simulink model "Marine_LocoMotive_UAV"  (R2018a)
settings: Solver=ode4  StartTime=0.0  StopTime=80  FixedStep=T  RelTol=1e-3
values from neighbouring files (symbols this model uses):
  a_11 = 0.05*m_b    (= 0.625)    [Marine_LocoMotive_UAV.m]
  a_33 = m_b    (= 12.5)    [Marine_LocoMotive_UAV.m]
  A_w = 1*1.5/2    (= 0.75)    [Marine_LocoMotive_UAV.m]
  A_w2 = 1*0.27/2    (= 0.135)    [Marine_LocoMotive_UAV.m]
  Ac = 0.0331    [Marine_LocoMotive_UAV.m]
  alpha_bar = pi/4    (= 0.785398163397)    [Marine_LocoMotive_UAV.m]
  Am = sysd.denominator{1}    [Marine_LocoMotive_UAV.m]
  Am1_LPF = sysd.denominator{1}    [Marine_LocoMotive_UAV.m]
  Am2_LPF = sysd.denominator{1}    [Marine_LocoMotive_UAV.m]
  Am_asw_LPF = sysd.denominator{1}    [Marine_LocoMotive_UAV.m]
  Am_coup_LPF = sysd.denominator{1}    [Marine_LocoMotive_UAV.m]
  Am_rdeL_LPF = sysd.denominator{1}    [Marine_LocoMotive_UAV.m]
  Am_reL_LPF = sysd.denominator{1}    [Marine_LocoMotive_UAV.m]
  Am_rref20_LPF = sysd.denominator{1}    [Marine_LocoMotive_UAV.m]
  Am_rref_LPF = sysd.denominator{1}    [Marine_LocoMotive_UAV.m]
  AmAlpha_LPF = sysd.denominator{1}    [Marine_LocoMotive_UAV.m]
  Amp_sf = 3    [Marine_LocoMotive_UAV.m]
  AmV_LPF = sysd.denominator{1}    [Marine_LocoMotive_UAV.m]
  AmZ_LPF = sysd.denominator{1}    [Marine_LocoMotive_UAV.m]
  b_11 = 0    [Marine_LocoMotive_UAV.m]
  b_33 = 2*m_b*omega_h    (= 27.5578302946)    [Marine_LocoMotive_UAV.m]
  Bm = sysd.numerator{1}    [Marine_LocoMotive_UAV.m]
  Bm1_LPF = sysd.numerator{1}    [Marine_LocoMotive_UAV.m]
  Bm2_LPF = sysd.numerator{1}    [Marine_LocoMotive_UAV.m]
  Bm_asw_LPF = sysd.numerator{1}    [Marine_LocoMotive_UAV.m]
  Bm_coup_LPF = sysd.numerator{1}    [Marine_LocoMotive_UAV.m]
  Bm_rdeL_LPF = sysd.numerator{1}    [Marine_LocoMotive_UAV.m]
  Bm_reL_LPF = sysd.numerator{1}    [Marine_LocoMotive_UAV.m]
  Bm_rref20_LPF = sysd.numerator{1}    [Marine_LocoMotive_UAV.m]
  Bm_rref_LPF = sysd.numerator{1}    [Marine_LocoMotive_UAV.m]
  BmAlpha_LPF = sysd.numerator{1}    [Marine_LocoMotive_UAV.m]
  BmV_LPF = sysd.numerator{1}    [Marine_LocoMotive_UAV.m]
  BmZ_LPF = sysd.numerator{1}    [Marine_LocoMotive_UAV.m]
  C_S = [5;9]*10^-3    [Marine_LocoMotive_UAV.m]
  Cd_u = 0.2    [Marine_LocoMotive_UAV.m]
  D_x = b_11 + D_s(1)    [Marine_LocoMotive_UAV.m]
  D_z = b_33 + D_s(2)    [Marine_LocoMotive_UAV.m]
  dc_M_p = 6.7    [Marine_LocoMotive_UAV.m]
  Delta_h = (A_im/A_b-0.5)*h_b    (= -0.0625)    [Marine_LocoMotive_UAV.m]
  eps_V = 0.1    [Marine_LocoMotive_UAV.m]
  epsilon_1 = 5    [Marine_LocoMotive_UAV.m]
  epsilon_e_u1 = 0.05    [Marine_LocoMotive_UAV.m]
  epsilon_w = 0    [Marine_LocoMotive_UAV.m]
  epsilon_w2 = pi    (= 3.14159265359)    [Marine_LocoMotive_UAV.m]
  g = 9.81    [Marine_LocoMotive_UAV.m]
  gamma_d_p = (2*0.3/0.03*2*0.2*12/4)/10    (= 2.4)    [Marine_LocoMotive_UAV.m]
  H = 10    [Marine_LocoMotive_UAV.m]
  h_b = 0.25    [Marine_LocoMotive_UAV.m]
  J_b = m_b*h_b*l_b/12    (= 0.208333333333)    [Marine_LocoMotive_UAV.m]
  J_u = 0.03    [Marine_LocoMotive_UAV.m]
  K = 40    [Marine_LocoMotive_UAV.m]
  k3 = 24    [Marine_LocoMotive_UAV.m]
  k4 = 0.8    [Marine_LocoMotive_UAV.m]
  k_w = omega_w^2/g    (= 0.123862835563)    [Marine_LocoMotive_UAV.m]
  k_w2 = omega_w2^2/g    (= 0.447144836384)    [Marine_LocoMotive_UAV.m]
  kd_a = 5.6    [Marine_LocoMotive_UAV.m]
  kd_r = 19.5    [Marine_LocoMotive_UAV.m]
  kd_t = 10    [Marine_LocoMotive_UAV.m]
  kd_x = 5    [Marine_LocoMotive_UAV.m]
  kd_z = 2    [Marine_LocoMotive_UAV.m]
  ki_a = 1.6    [Marine_LocoMotive_UAV.m]
  ki_r = 9    [Marine_LocoMotive_UAV.m]
  ki_T = 12    [Marine_LocoMotive_UAV.m]
  ki_x = 1.2    [Marine_LocoMotive_UAV.m]
  ki_z = 1    [Marine_LocoMotive_UAV.m]
  kp_a = 9.6    [Marine_LocoMotive_UAV.m]
  kp_r = 45    [Marine_LocoMotive_UAV.m]
  kp_t = 20    [Marine_LocoMotive_UAV.m]
  kp_T = 25    [Marine_LocoMotive_UAV.m]
  kp_x = 7    [Marine_LocoMotive_UAV.m]
  kp_z = 3    [Marine_LocoMotive_UAV.m]
  L = 0.2    [Marine_LocoMotive_UAV.m]
  l_b = 0.8    [Marine_LocoMotive_UAV.m]
  Lc_0 = 7    [Marine_LocoMotive_UAV.m]
  LIMIT_CMD_PITCH = 45*pi/180    (= 0.785398163397)    [Marine_LocoMotive_UAV.m]
  LIMIT_uCMD_HEIGHT = 3.5*K    (= 140)    [Marine_LocoMotive_UAV.m]
  m_b = rho_w*Vol_b/4    (= 12.5)    [Marine_LocoMotive_UAV.m]
  m_u = 1.8    [Marine_LocoMotive_UAV.m]
  min_sf = 5    [Marine_LocoMotive_UAV.m]
  nu_w = 1.787*10^-6    (= 1.787e-06)    [Marine_LocoMotive_UAV.m]
  omega_w = 2*pi/T_w    (= 1.10231321179)    [Marine_LocoMotive_UAV.m]
  omega_w2 = 2*pi/T_w2    (= 2.09439510239)    [Marine_LocoMotive_UAV.m]
  r_0 = sqrt( (X0_b(1) - X0_u(1))^2 +(X0_b(2) - X0_u(2))^2 )    [Marine_LocoMotive_UAV.m]
  r_bar = Lc_0-0.3    (= 6.7)    [Marine_LocoMotive_UAV.m]
  r_min = (zu_bar-H)-0.2    [Marine_LocoMotive_UAV.m]
  rho_a = 1.225    [Marine_LocoMotive_UAV.m]
  rho_w = 1000    [Marine_LocoMotive_UAV.m]
  T = 1/500    (= 0.002)    [Marine_LocoMotive_UAV.m]
  T_init = 10    [Marine_LocoMotive_UAV.m]
  Theta0 = 0*atan2(V_bar*D_x*cos(alpha_bar_0),V_bar*D_x*sin(alpha_bar_0)+m_u*g*cos(alpha_bar_0))    [Marine_LocoMotive_UAV.m]
  u_s = w_dir*A_w^2*omega_w*k_w*exp(2*k_w*(-Delta_h/2))    [Marine_LocoMotive_UAV.m]
  u_s2 = w_dir2*A_w2^2*omega_w2*k_w2*exp(2*k_w2*(-Delta_h/2))    [Marine_LocoMotive_UAV.m]
  u_t = -1*0.5*1    (= -0.5)    [Marine_LocoMotive_UAV.m]
  u_w = 0*0.2    (= 0)    [Marine_LocoMotive_UAV.m]
  V0_b = [u_t+u_w+u_s+v_x_w, v_z_w]    [Marine_LocoMotive_UAV.m]
  V0_u = [0 0]    [Marine_LocoMotive_UAV.m]
  V_bar = 4    [Marine_LocoMotive_UAV.m]
  Vol_b = A_b*l_b    (= 0.05)    [Marine_LocoMotive_UAV.m]
  w_dir = 1    [Marine_LocoMotive_UAV.m]
  w_dir2 = 1    [Marine_LocoMotive_UAV.m]
  X0_b = [0,H-Delta_h]    [Marine_LocoMotive_UAV.m]
  X0_u = X0_b + [3 3]    [Marine_LocoMotive_UAV.m]
  zu_bar = X0_b(2) + Lc_0*sin(alpha_bar_0)    [Marine_LocoMotive_UAV.m]
undefined symbols (not defined in the file or in its folder): Am_HPF, Am_LPF, Am_LPF2, an1, an1_v, an2, an3, Bm_HPF, Bm_LPF, Bm_LPF2, bn1, bn1_v, bn2, bn3, DiscIntNeverNeededParam, F, Light, magnitude, MIL, OMEGA_FILTER_OUTER, R_b, Tc, Tg, Tn, Ts, Tsc, Tz, X_GPS_offset
libraries: simulink x50, simulink_extras x9, aerolibwind2 x2
(part 2 of 6)

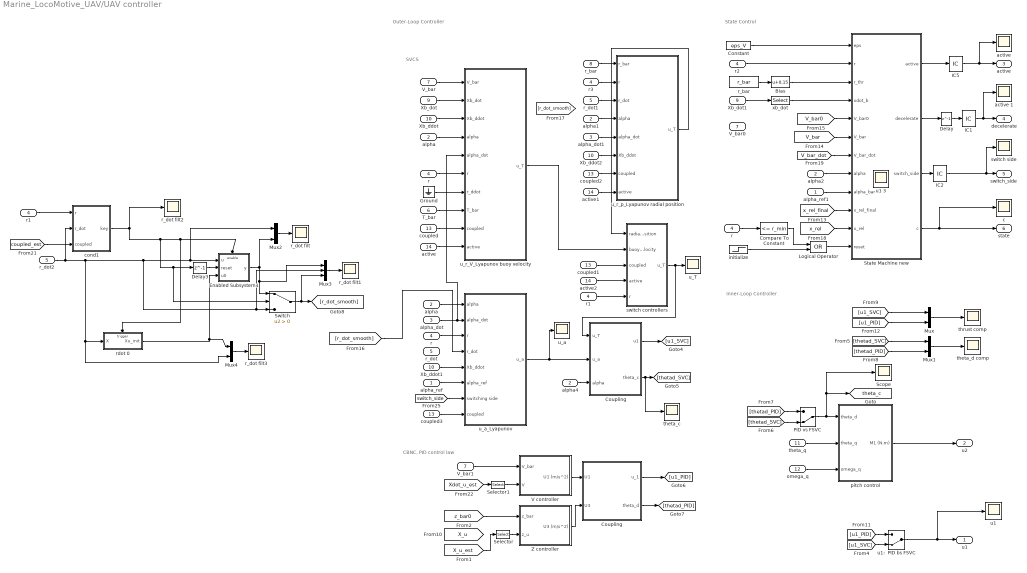
== system Marine_LocoMotive_UAV/UAV controller ==
  note: State Control
  note: Inner-Loop Controller
  note: Outer-Loop Controller
  note: CBNC, PID control law
  note: SVCS
  alpha_ref : Inport
  alpha : Inport  Port=2
  alpha_dot : Inport  Port=3
  r : Inport  Port=4
  r_dot : Inport  Port=5
  T_bar : Inport  Port=6
  V_bar : Inport  Port=7
  r_bar : Inport  Port=8
  Xb_dot : Inport  Port=9
  Xb_ddot : Inport  Port=10
  theta_q : Inport  Port=11
  omega_q : Inport  Port=12
  coupled : Inport  Port=13
  active : Inport  Port=14
  " active " : Scope
  " active 1" : Scope
  " c " : Scope
  " r" : InportShadow  Port=4
  " r1" : InportShadow  Port=4
  Bias : Bias  Bias=0.15
  Compare To Constant : simulink/Logic and Bit Operations/Compare To Constant  relop=<=  const=r_min  OutDataTypeStr=boolean
  Constant : Constant  Value=eps_V
  Coupling : Subsystem
  "Coupling " : Subsystem
  Delay : Delay  DelayLength=1  InitialCondition=0
  Delay3 : Delay  DelayLength=1  InitialCondition=0
  Enabled Subsystem1 : Subsystem  TreatAsAtomicUnit=on
  Ground : Ground
  IC1 : InitialCondition  Value=0
  IC2 : InitialCondition  Value=0
  IC5 : InitialCondition  Value=0
  Logical Operator : Logic  Operator=OR  AllPortsSameDT=off  OutDataTypeStr=boolean
  Mux{,1..2,4} (4 alike) : Mux  Inputs=2
  Mux3 : Mux  Inputs=3
  PID vs FSVC : ManualSwitch  CurrentSetting=0
  Scope : Scope
  Selector : Selector  InputPortWidth=2  IndexOptions=Index vector (dialog)  Indices=2  OutputSizes=1
  Selector1 : Selector  InputPortWidth=2  IndexOptions=Index vector (dialog)  Indices=1  OutputSizes=1
  State Machine new : MATLAB Function  TreatAsAtomicUnit=on
  Switch : Switch  Criteria=u2 > Threshold
  V controller : Subsystem
  V_bar0 : InportShadow  Port=7
  V_bar1 : InportShadow  Port=7
  Xb_ddot1 : InportShadow  Port=10
  Xb_ddot2 : InportShadow  Port=10
  Xb_dot1 : InportShadow  Port=9
  Z controller : Subsystem
  active1 : InportShadow  Port=14
  active2 : InportShadow  Port=14
  "alpha " : InportShadow  Port=2
  alpha1 : InportShadow  Port=2
  alpha2 : InportShadow  Port=2
  alpha4 : InportShadow  Port=2
  alpha_dot1 : InportShadow  Port=3
  alpha_ref1 : InportShadow
  cond1 : Subsystem
  coupled1 : InportShadow  Port=13
  coupled2 : InportShadow  Port=13
  coupled3 : InportShadow  Port=13
  initialize : Step  Time=T_init  Before=1  After=0  SampleTime=0
  pitch control : Subsystem
  "r " : InportShadow  Port=4
  r1 : InportShadow  Port=4
  r2 : InportShadow  Port=4
  r3 : InportShadow  Port=4
  "r_bar " : Constant  Value=r_bar
  r_dot filt{,1..3} (4 alike) : Scope
  r_dot1 : InportShadow  Port=5
  r_dot2 : InportShadow  Port=5
  rdot 0 : Subsystem  TreatAsAtomicUnit=on
  switch controllers : Subsystem
  "switch side  " : Scope
  "theta_c " : Scope
  theta_d comp : Scope
  thrust comp : Scope
  "u1 " : Scope
  u1 3 : Scope
  u1:  PID bs FSVC : ManualSwitch  CurrentSetting=0
  u_T : Scope
  u_a : Scope
  u_a_Lyapunov : Subsystem
  u_r_V_Lyapunov buoy velocity : Subsystem
  u_r_p_Lyapunov radial position : Subsystem
  xb_dot : Selector  InputPortWidth=2  IndexOptions=Index vector (dialog)  Indices=1  OutputSizes=1
  u1 : Outport
  u2 : Outport  Port=2
  " active" : Outport  Port=3
  " decelerate" : Outport  Port=4
  " switch_side" : Outport  Port=5
  state : Outport  Port=6
  tag scope: theta_c=global
  wires:
  theta_q/1 -> pitch control/2(theta_q)
  omega_q/1 -> pitch control/3(omega_q)
  pitch control/1(M1 (N.m)) -> u2/1
  alpha4/1 -> "Coupling "/3(alpha)
  PID vs FSVC/1 -> Scope/1, [theta_c], pitch control/1(theta_d)
  u1:  PID bs FSVC/1 -> "u1 "/1, u1/1
  alpha/1 -> u_r_V_Lyapunov buoy velocity/4(alpha)
  T_bar/1 -> u_r_V_Lyapunov buoy velocity/8(T_bar)
  V_bar/1 -> u_r_V_Lyapunov buoy velocity/1(V_bar)
  Xb_dot/1 -> u_r_V_Lyapunov buoy velocity/2(Xb_dot)
  Xb_ddot/1 -> u_r_V_Lyapunov buoy velocity/3(Xb_ddot)
  "alpha "/1 -> u_a_Lyapunov/1(alpha)
  Xb_ddot1/1 -> u_a_Lyapunov/5(Xb_ddot)
  alpha_ref/1 -> u_a_Lyapunov/6(alpha_ref)
  alpha_dot/1 -> u_r_V_Lyapunov buoy velocity/5(alpha_dot), u_a_Lyapunov/2("alpha_dot ")
  [z_bar0] -> Z controller/1(z_bar)
  Selector/1 -> Z controller/2(z_u)
  [X_u_est] -> Selector/1
  V_bar1/1 -> V controller/1(V_bar)
  [Xdot_u_est] -> Selector1/1
  Selector1/1 -> V controller/2(V)
  V controller/1(U1 (m/s^2)) -> Coupling/1(U1)
  Z controller/1(U3 (m/s^2)) -> Coupling/2(U3)
  Mux/1 -> thrust comp/1
  Mux1/1 -> theta_d comp/1
  [thetad_SVC] -> Mux1/1
  [u1_SVC] -> u1:  PID bs FSVC/2
  u_a_Lyapunov/1(u_a) -> u_a/1, "Coupling "/2(u_a)
  Xb_dot1/1 -> xb_dot/1
  [V_bar0] -> State Machine new/5(V_bar0)
  xb_dot/1 -> State Machine new/4(xdot_b)
  Constant/1 -> State Machine new/1(eps)
  State Machine new/1(active) -> IC5/1
  State Machine new/4(c) -> state/1, " c "/1
  IC5/1 -> " active "/1, " active"/1
  Coupling/1(u_1) -> [u1_PID]
  Coupling/2(theta_d) -> [thetad_PID]
  "Coupling "/1(u1) -> [u1_SVC]
  [thetad_SVC] -> PID vs FSVC/2
  [thetad_PID] -> PID vs FSVC/1
  [thetad_PID] -> Mux1/2
  [u1_SVC] -> Mux/1
  [u1_PID] -> u1:  PID bs FSVC/1
  [u1_PID] -> Mux/2
  "Coupling "/2(theta_c) -> "theta_c "/1, [thetad_SVC]
  r_bar/1 -> u_r_p_Lyapunov radial position/1("r_bar ")
  r/1 -> Compare To Constant/1
  Compare To Constant/1 -> Logical Operator/1
  initialize/1 -> Logical Operator/2
  active/1 -> u_r_V_Lyapunov buoy velocity/10(active)
  coupled/1 -> u_r_V_Lyapunov buoy velocity/9(coupled)
  Ground/1 -> u_r_V_Lyapunov buoy velocity/7(r_ddot)
  [r_dot_smooth] -> u_a_Lyapunov/4(r_dot)
  "r "/1 -> u_r_V_Lyapunov buoy velocity/6(r)
  " r"/1 -> u_a_Lyapunov/3(r)
  r3/1 -> u_r_p_Lyapunov radial position/2(r)
  r_dot1/1 -> u_r_p_Lyapunov radial position/3(r_dot)
  alpha1/1 -> u_r_p_Lyapunov radial position/4(alpha)
  alpha_dot1/1 -> u_r_p_Lyapunov radial position/5(alpha_dot)
  Xb_ddot2/1 -> u_r_p_Lyapunov radial position/6(Xb_ddot)
  active1/1 -> u_r_p_Lyapunov radial position/8(active)
  "r_bar "/1 -> Bias/1
  coupled2/1 -> u_r_p_Lyapunov radial position/7(coupled)
  switch controllers/1(u_T) -> "Coupling "/1(u_T), u_T/1
  u_r_V_Lyapunov buoy velocity/1(u_T) -> switch controllers/2(buoy velocity)
  coupled1/1 -> switch controllers/3(coupled)
  active2/1 -> switch controllers/4(active)
  u_r_p_Lyapunov radial position/1(u_T) -> switch controllers/1(radial position)
  State Machine new/2(decelerate) -> Delay/1
  IC1/1 -> " active 1"/1, " decelerate"/1
  alpha_ref1/1 -> State Machine new/9(alpha_bar)
  alpha2/1 -> State Machine new/8(alpha)
  State Machine new/3(switch_side) -> IC2/1
  IC2/1 -> "switch side  "/1, " switch_side"/1
  Logical Operator/1 -> State Machine new/12(reset)
  r1/1 -> switch controllers/5(r)
  [x_rel_final] -> State Machine new/10(x_rel_final)
  [switch_side] -> u_a_Lyapunov/7(switching side)
  Mux2/1 -> r_dot filt/1
  Enabled Subsystem1/1(y) -> Mux2/2, Mux3/1, Switch/1
  Switch/1 -> Mux3/3, [r_dot_smooth]
  Mux3/1 -> r_dot filt1/1
  [coupled_est] -> cond1/3(coupled)
  coupled3/1 -> u_a_Lyapunov/8(coupled)
  r_dot2/1 -> cond1/2(r_dot), Enabled Subsystem1/1(u), Mux2/1, Mux3/2, Switch/3, rdot 0/1(X), Mux4/2
  Mux4/1 -> r_dot filt3/1
  rdot 0/1(Xu_init) -> Mux4/1, Enabled Subsystem1/3(u0)
  " r1"/1 -> cond1/1(r)
  cond1/1(key) -> Delay3/1, Switch/2, rdot 0/Trigger, Enabled Subsystem1/Enable, r_dot filt2/1
  Delay3/1 -> Enabled Subsystem1/2(reset)
  [x_rel] -> State Machine new/11(x_rel)
  [V_bar] -> State Machine new/6(V_bar)
  Bias/1 -> State Machine new/3(r_thr)
  [V_bar_dot] -> State Machine new/7(V_bar_dot)
  Delay/1 -> IC1/1
  r2/1 -> State Machine new/2(r)

== system Marine_LocoMotive_UAV/Wind model ==
  Bias : Bias  Bias=0.05
  Discrete Wind Gust Model : aerolibwind2/Discrete Wind Gust Model  units=Metric (MKS)  Gx=on  Gy=off  Gz=off  t_0=1  d_m=[1 1 80]  v_m=V_w
      settings: SourceProductName=Aerospace Blockset
  Dryden Wind Turbulence Model (Continuous (+q +r)) : aerolibwind2/Dryden Wind Turbulence Model  (Continuous (+q -r))  Commented=on  units=Metric (MKS)  spec=MIL-F-8785C  model=Continuous Dryden (+q +r)  W20=20  Wdeg=30  TurbProb=10^-2 - Light  L_high=533.4  Wingspan=1.5  ts=0.02  Seed=[11341 23342 13423 13344]  T_on=on
      settings: SourceProductName=Aerospace Blockset
  From25 : From  Commented=on  GotoTag=X_u  TagVisibility=global
  From3 : From  Commented=on  GotoTag=DCM_b2e  TagVisibility=global
  Gain : Gain  Commented=on
  Math Function1 : Math  Commented=on  Operator=transpose  SaturateOnIntegerOverflow=on
  N3 : Scope
  Selector1 : Selector  InputPortWidth=3  IndexOptions=Index vector (dialog)  Indices=[1 3]  OutputSizes=1
  Selector2 : Selector  Commented=on  InputPortWidth=3  IndexOptions=Index vector (dialog)  Indices=2  OutputSizes=1
  Selector6 : Selector  Commented=on  InputPortWidth=2  IndexOptions=Index vector (dialog)  Indices=2  OutputSizes=1
  Zero-Order Hold : ZeroOrderHold  SampleTime=-1
  magnitude : Subsystem
  V_wind : Outport
  omega_wind : Outport  Port=2
  wires:
  Selector6/1 -> Gain/1
  Gain/1 -> Dryden Wind Turbulence Model (Continuous (+q +r))/1
  Bias/1 -> Dryden Wind Turbulence Model (Continuous (+q +r))/2, Discrete Wind Gust Model/1
  Math Function1/1 -> Dryden Wind Turbulence Model (Continuous (+q +r))/3
  From3/1 -> Math Function1/1
  Dryden Wind Turbulence Model (Continuous (+q +r))/2 -> Selector2/1
  magnitude/1(Out1) -> Bias/1
  From25/1 -> Selector6/1
  [Xdot_u] -> magnitude/1(In1)
  Discrete Wind Gust Model/1 -> Selector1/1
  Selector1/1 -> Zero-Order Hold/1
  Selector2/1 -> omega_wind/1
  Zero-Order Hold/1 -> N3/1, V_wind/1

== system Marine_LocoMotive_UAV/Preprocessing Unit/Alpha_bar ==
  note: x_rel true
  note: Key to specify "front" or "rear" configuration.
  note: find desired x_rel and z_rel for the UAV:
      | x_rel_des = sqrt(r_bar^2 - (zu_bar-zb)^2)
      |
      | Note that the sign of x_rel is still anbiguous at this stage
  note: 1- Calculate alpha_bar based on x_rel and z_rel
  note: Z bar calculation during switching side mode:
      | (the UAV elevation changes from the reference hold).
      | This signal is used for monitoring purpose (not used by the controller)
  zb : Inport
  r_bar : Inport  Port=2
  zq_bar : Inport  Port=3
  alpha : Inport  Port=4
  decelerate : Inport  Port=5
  switch side : Inport  Port=6
  "  " : Trigonometry
  Delay1 : Delay  DelayLength=1
  Logical Operator1 : Logic  AllPortsSameDT=off  OutDataTypeStr=boolean
  Math Function : Math  Operator=magnitude^2  SaturateOnIntegerOverflow=on
  Math Function2 : Math  Operator=magnitude^2  SaturateOnIntegerOverflow=on
  Mux1 : Mux  Inputs=2
  Mux2 : Mux  Inputs=2
  Product2 : Product
  Sqrt : Sqrt  SaturateOnIntegerOverflow=on
  Sum : Sum  Inputs=|+-
  Sum1 : Sum  Inputs=|+-
  Sum2 : Sum  Inputs=|++
  Switch1 : Switch  Criteria=u2 > Threshold
  Switch2 : Switch  Criteria=u2 > Threshold
  Unary Minus : UnaryMinus
  "alpha_bar " : Trigonometry  Operator=atan2
  decelerate2 : InportShadow  Port=5
  has moved past the buoy1 : simulink/Logic and Bit Operations/Compare To Constant  relop=>  const=pi/2  OutDataTypeStr=boolean
  r_bar1 : InportShadow  Port=2
  smooth switch : Subsystem
  x_rel des : Scope
  x_rel_amb : Scope
  z_bar_ss : Scope
  z_rel : Scope
  z_rel1 : Scope
  zb1 : InportShadow
  zq_bar1 : InportShadow  Port=3
  alpha_bar : Outport
  x_rel_bar : Outport  Port=2
  z_bar : Outport  Port=3
  tag scope: alpha_bar_step=global, x_rel=global, x_rel_amb=global, x_rel_final=global
  wires:
  [x_rel] -> "alpha_bar "/2  "x_rel"
  Sum/1 -> z_rel/1, [z_rel], Math Function2/1  "z_rel"
  zb/1 -> Sum/2
  Math Function2/1 -> Sum1/2
  zq_bar/1 -> Sum/1
  r_bar/1 -> Math Function/1
  Math Function/1 -> Sum1/1
  Sum1/1 -> Sqrt/1
  [x_rel_amb] -> Switch1/3, smooth switch/1(u 1), Unary Minus/1  "x_rel_des"
  alpha/1 -> has moved past the buoy1/1
  [z_rel] -> "alpha_bar "/1
  decelerate/1 -> Logical Operator1/2
  has moved past the buoy1/1 -> Logical Operator1/1
  Logical Operator1/1 -> Delay1/1
  switch side/1 -> Switch2/2
  zq_bar1/1 -> Switch2/3
  Switch2/1 -> Mux2/2, z_bar/1
  zb1/1 -> Sum2/1
  Sum2/1 -> Mux2/1, Switch2/1
  [alpha_bar_step] -> "  "/1
  "  "/1 -> Product2/1
  r_bar1/1 -> Product2/2
  Product2/1 -> Sum2/2
  Sqrt/1 -> x_rel_amb/1, [x_rel_amb]  "x_rel_des"
  Delay1/1 -> [rear]
  "alpha_bar "/1 -> z_rel1/1, alpha_bar/1, [alpha_bar_step]
  smooth switch/1(y) -> Mux1/1, x_rel_bar/1, [x_rel]  "x_rel"
  Mux2/1 -> z_bar_ss/1
  decelerate2/1 -> Switch1/2, smooth switch/3(switch)
  Switch1/1 -> Mux1/2, [x_rel_final]
  Unary Minus/1 -> smooth switch/2(u 2), Switch1/1
  Mux1/1 -> x_rel des/1

== system Marine_LocoMotive_UAV/Preprocessing Unit/Buoy immersed volume estimation ==
  note: Expected Immersed Volume (m^3)
      | (based on exact damping coefficient)
  note: Mean Immersed Volume (m^3)
      | (based on estimated damping coefficient)
  Constant : Constant  Value=(m_b+m_u)/rho_w
  Constant1 : Constant  Value=(m_b+m_u)/rho_w
  Constant2 : Constant  Value=rho_w*g
  Constant3 : Constant  Value=rho_w*g
  Constant4 : Constant  Value=0
  Constant5 : Constant  Value=Vol_b
  Constant6 : Constant
  Constant7 : Constant
  D11 1 : Scope
  D11 3 : Scope
  D_1 : Selector  NumberOfDimensions=2  InputPortWidth=2  IndexOptions=Index vector (dialog),Index vector (dialog)  Indices=1,1  OutputSizes=1,1
  D_21 : Selector  NumberOfDimensions=2  InputPortWidth=2  IndexOptions=Index vector (dialog),Index vector (dialog)  Indices=2,1  OutputSizes=1,1
  Dead Zone : DeadZone  Commented=on  LowerValue=80*pi/180  UpperValue=100*pi/180  SaturateOnIntegerOverflow=on
  Divide : Product  Inputs=*/
  IC1 : InitialCondition  Value=Delta_h*l_b*h_b + l_b*h_b^2/2
  Mux2 : Mux  Inputs=2
  Product : Product  Inputs=*/
  Product1 : Product  Inputs=*/*
  Product2 : Product  Inputs=*/
  Product3 : Product  Inputs=*/*
  Saturation1 : Saturate  UpperLimit=inf  LowerLimit=0.1*pi/180
  Saturation2 : Saturate  UpperLimit=60*pi/180  LowerLimit=0.1*pi/180
  Sum1 : Sum  Inputs=|++
  Sum2 : Sum  Inputs=|+-
  Sum3 : Sum  Inputs=|++
  Sum4 : Sum  Inputs=|+-
  Trigonometric Function : Trigonometry  Operator=tan
  Trigonometric Function1 : Trigonometry  Operator=tan
  V_immersed ratio : Scope
  Vol_im_expected : Outport
  Vol_im_mean : Outport  Port=2
  wires:
  [V_r_bar] -> Product1/1
  Constant1/1 -> Sum3/1
  Sum2/1 -> D11 1/1, Product1/3
  Constant3/1 -> Product3/2
  Constant4/1 -> Sum4/1
  D_21/1 -> Sum2/1
  [D_123] -> D_1/1
  [D_123] -> D_21/1
  D_1/1 -> Product/1
  Product2/1 -> Sum4/2
  Saturation2/1 -> Trigonometric Function1/1
  Product3/1 -> Sum3/2
  Product1/1 -> Sum1/2
  Sum4/1 -> D11 3/1, Product3/3
  Constant/1 -> Sum1/1
  [V_r_bar] -> Product3/1
  Product/1 -> Sum2/2
  Saturation1/1 -> Trigonometric Function/1
  [theta_bar] -> Saturation1/1
  Constant2/1 -> Product1/2
  [theta_bar] -> Saturation2/1
  Sum3/1 -> IC1/1
  Constant7/1 -> Product/2
  [D11_bar] -> Product2/1
  Constant6/1 -> Product2/2
  Sum1/1 -> Mux2/1, Vol_im_expected/1
  IC1/1 -> Mux2/2, Vol_im_mean/1
  Divide/1 -> V_immersed ratio/1
  Constant5/1 -> Divide/2
  Mux2/1 -> Divide/1

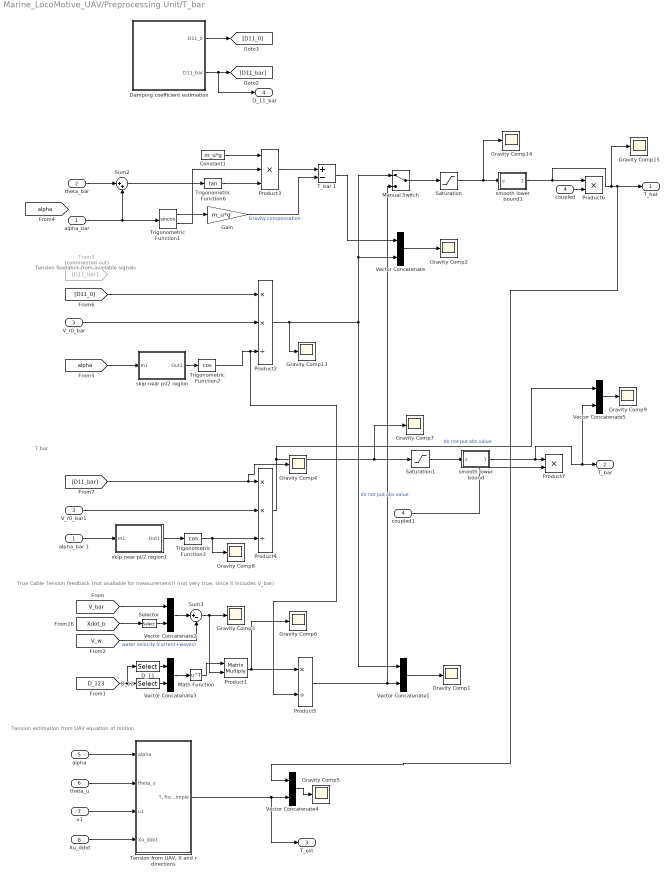
== system Marine_LocoMotive_UAV/Preprocessing Unit/T_bar  ==
  note: Tension feadabck from available signals
  note: True Cable Tension feedback (not available for measurement!) (not very true, since it includes V_bar)
  note: T bar
  note: Tension estimation from UAV equation of motion
  "alpha_bar " : Inport
  theta_bar : Inport  Port=2
  V_r0_bar : Inport  Port=3
  coupled : Inport  Port=4
  alpha : Inport  Port=5
  theta_u : Inport  Port=6
  u1 : Inport  Port=7
  Xu_ddot : Inport  Port=8
  Constant1 : Constant  Value=m_u*g
  D_11 : Selector  NumberOfDimensions=2  InputPortWidth=2  IndexOptions=Index vector (dialog),Index vector (dialog)  Indices=1,1  OutputSizes=1,1
  D_12 : Selector  NumberOfDimensions=2  InputPortWidth=2  IndexOptions=Index vector (dialog),Index vector (dialog)  Indices=1,2  OutputSizes=1,1
  Damping coefficient estimation : Subsystem
  From3 : From  Commented=on  GotoTag=D11_bar  TagVisibility=global
  Gain : Gain  Gain=m_u*g
  Gravity Comp{1..9,13..15} (12 alike) : Scope
  Manual Switch : ManualSwitch
  Math Function : Math  Operator=transpose  SaturateOnIntegerOverflow=on
  Product1 : Product  Multiplication=Matrix(*)
  Product2 : Product  Inputs=**/
  Product3 : Product  Inputs=***
  Product4 : Product  Inputs=**/
  Product5 : Product  Inputs=*/
  Product6 : Product
  Product7 : Product
  Saturation : Saturate  UpperLimit=inf  LowerLimit=epsilon_1
  Saturation1 : Saturate  UpperLimit=inf  LowerLimit=0
  Selector : Selector  InputPortWidth=2  IndexOptions=Index vector (dialog)  Indices=2  OutputSizes=1
  Sum2 : Sum  Inputs=|++
  Sum3 : Sum  Inputs=|+-
  T_bar 1 : Sum  Inputs=+-
  "Tension from UAV, X and r directions" : Subsystem
  Trigonometric Function1 : Trigonometry  Operator=sincos
  Trigonometric Function2 : Trigonometry  Operator=cos
  Trigonometric Function3 : Trigonometry  Operator=cos
  Trigonometric Function6 : Trigonometry  Operator=tan
  V_r0_bar1 : InportShadow  Port=3
  Vector Concatenate{,1..5} (6 alike) : Concatenate
  alpha_bar 1 : InportShadow
  coupled1 : InportShadow  Port=4
  skip near pi/2 region : Subsystem
  skip near pi/2 region1 : Subsystem
  smooth lower bound : Subsystem
  smooth lower bound1 : Subsystem
  T_hat : Outport
  T_bar : Outport  Port=2
  T_est : Outport  Port=3
  D_11_bar : Outport  Port=4
  wires:
  "alpha_bar "/1 -> Sum2/2, Trigonometric Function1/1
  Trigonometric Function1/1 -> Gain/1
  Gain/1 -> T_bar 1/2  "Gravity compensation"
  theta_bar/1 -> Sum2/1
  Sum2/1 -> Trigonometric Function6/1
  Vector Concatenate1/1 -> Gravity Comp1/1
  [D11_0] -> Product2/1
  Vector Concatenate/1 -> Gravity Comp2/1
  Constant1/1 -> Product3/1
  Trigonometric Function1/2 -> Product3/2
  Trigonometric Function6/1 -> Product3/3
  Product3/1 -> T_bar 1/1
  [D_123] -> D_11/1, D_12/1
  D_11/1 -> Vector Concatenate3/1
  [Xdot_b] -> Selector/1
  Sum3/1 -> Product1/2, Gravity Comp3/1
  Vector Concatenate2/1 -> Sum3/1
  [V_w] -> Sum3/2  "water velocity (current+waves)"
  Product1/1 -> Gravity Comp6/1, Product5/1
  Product5/1 -> Manual Switch/2, Vector Concatenate1/2
  Manual Switch/1 -> Saturation/1
  T_bar 1/1 -> Vector Concatenate/1
  Trigonometric Function2/1 -> Product5/2, Product2/3
  [V_bar] -> Vector Concatenate2/1
  Selector/1 -> Vector Concatenate2/2
  D_12/1 -> Vector Concatenate3/2
  Vector Concatenate3/1 -> Math Function/1
  Math Function/1 -> Product1/1
  alpha_bar 1/1 -> skip near pi/2 region1/1(In1)
  [D11_bar] -> Product4/1, Gravity Comp4/1
  Trigonometric Function3/1 -> Gravity Comp8/1, Product4/3
  Saturation/1 -> Gravity Comp14/1, smooth lower bound1/1(u)
  coupled/1 -> Product6/2
  Saturation1/1 -> smooth lower bound/1(u)
  skip near pi/2 region1/1(Out1) -> Trigonometric Function3/1
  theta_u/1 -> "Tension from UAV, X and r directions"/2(theta_u)
  alpha/1 -> "Tension from UAV, X and r directions"/1(alpha)
  Xu_ddot/1 -> "Tension from UAV, X and r directions"/4(Xu_ddot)
  u1/1 -> "Tension from UAV, X and r directions"/3(u1)
  Vector Concatenate4/1 -> Gravity Comp5/1
  Damping coefficient estimation/1(D11_0) -> [D11_0]
  Damping coefficient estimation/2(D11_bar) -> [D11_bar], D_11_bar/1
  coupled1/1 -> Product7/2
  smooth lower bound/1(sat(u)) -> Vector Concatenate5/2, T_bar/1, Product7/1
  V_r0_bar1/1 -> Product4/2
  Product4/1 -> Gravity Comp7/1, Saturation1/1, Vector Concatenate5/1  "do not put abs value"
  Vector Concatenate5/1 -> Gravity Comp9/1
  smooth lower bound1/1(sat(u)) -> Gravity Comp15/1, Vector Concatenate4/1, T_hat/1, Product6/1
  "Tension from UAV, X and r directions"/1("T, from x simple") -> T_est/1, Vector Concatenate4/2
  Product2/1 -> Manual Switch/1, Vector Concatenate/2, Vector Concatenate1/1, Gravity Comp13/1  "do not put abs value"
  V_r0_bar/1 -> Product2/2
  [alpha] -> skip near pi/2 region/1(In1)
  skip near pi/2 region/1(Out1) -> Trigonometric Function2/1

== system Marine_LocoMotive_UAV/Preprocessing Unit/Theta_bar  ==
  "alpha_bar " : Inport
  V_r0_bar : Inport  Port=2
  D11_bar : Inport  Port=3
  switch side1 : Inport  Port=4
  Add : Sum
  Constant : Constant  Value=alpha_bar
  D_11 : Selector  NumberOfDimensions=2  InputPortWidth=2  IndexOptions=Index vector (dialog),Index vector (dialog)  Indices=1,1  OutputSizes=1,1
  Gain : Gain  Gain=m_u*g
  Mux : Mux  Inputs=2
  Product1 : Product
  Product2 : Product  Inputs=**
  Product3 : Product
  Scope : Scope
  Switch : Switch  Criteria=u2 > Threshold
  Trigonometric Function3 : Trigonometry  Operator=sincos
  "theta_bar " : Trigonometry  Operator=atan2
  theta_bar : Outport
  wires:
  "theta_bar "/1 -> theta_bar/1
  "alpha_bar "/1 -> Switch/3
  Product1/1 -> "theta_bar "/1  "dy"
  Add/1 -> "theta_bar "/2  "dx"
  Product2/1 -> Add/1
  Trigonometric Function3/1 -> Product2/1
  Trigonometric Function3/2 -> Product1/2, Gain/1
  Gain/1 -> Add/2
  [D_123] -> D_11/1
  V_r0_bar/1 -> Product3/2
  Product3/1 -> Product2/2, Product1/1
  D11_bar/1 -> Mux/2, Product3/1
  Mux/1 -> Scope/1
  D_11/1 -> Mux/1
  switch side1/1 -> Switch/2
  Switch/1 -> Trigonometric Function3/1
  Constant/1 -> Switch/1

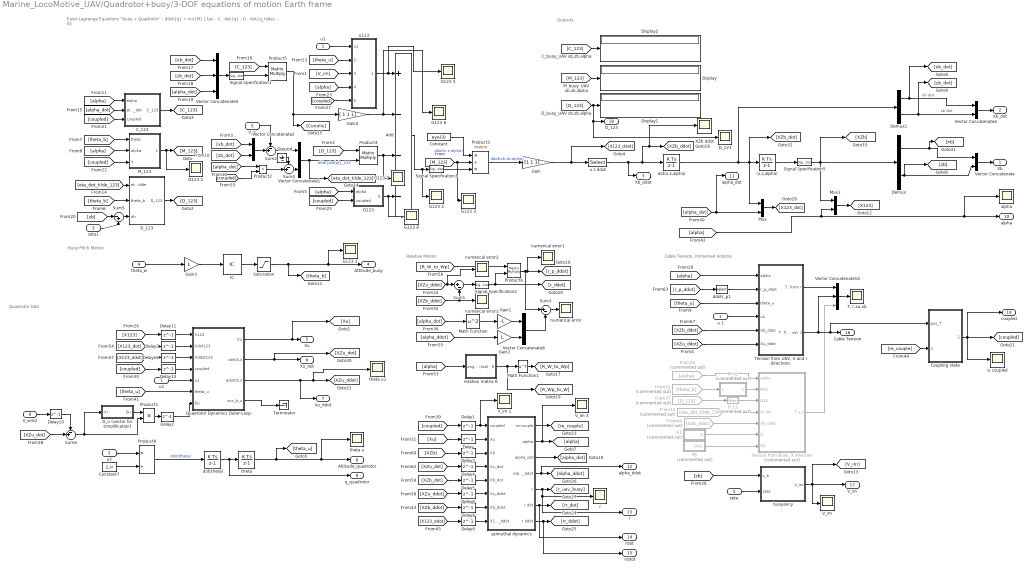
== system Marine_LocoMotive_UAV/Quadrotor+buoy/3-DOF equations of motion Earth frame ==
  note: Relative Motion
  note: Outputs
  note: Buoy Pitch Motion
  note: Cable Tension, Immersed Volume
  note: Quadrotor UAV
  note: Euler-Lagrange Equations "Buoy + Quadrotor" : ddot{q} = inv{M} [ tau - C . dot{q} - D . dot{q_tilde} - G]
  u1 : Inport
  u2 : Inport  Port=2
  zeta : Inport  Port=3
  theta_w : Inport  Port=4
  V_w : Inport  Port=5
  V_wind : Inport  Port=6
  "  r   " : Scope
  (x,z,alpha) : DiscreteIntegrator  InitialCondition=[pos_b_ini]  SampleTime=-1  ICPrevOutput=DiscIntNeverNeededParam  ICPrevScaledInput=DiscIntNeverNeededParam
  Add : Sum  Inputs=+---
  C_123 : Subsystem
  Constant : Constant  Value=eye(3)
  Constant7 : Constant  Value=J_u
  Coupling state : Subsystem
  D_12 : Selector  Commented=on  NumberOfDimensions=2  InputPortWidth=3  IndexOptions=Starting index (dialog),Starting index (dialog)  Indices=1,1  OutputSizes=2,2
  D_123 : Subsystem
  "D_123   " : Scope
  D_u (vector for simplification) : Subsystem
  Delay{,1,3..9,11..13} (12 alike) : Delay  DelayLength=1
  Delay10 : Delay  DelayLength=1  InitialCondition=[0 0]
  Delay2 : Delay  DelayLength=1  InitialCondition=[0 0]
  Demux : Demux  Outputs=2
  Demux1 : Demux  Outputs=2
  Display : Display
  Display1 : Display
  Display2 : Display
  FB : Subsystem  Commented=on
  From32 : From  Commented=on  GotoTag=eta_dot_tilde_12
  From34 : From  Commented=on  GotoTag=alpha
  From37 : From  Commented=on  GotoTag=D_123
  From44 : From  Commented=on  GotoTag=XZb_ddot
  From51 : From  Commented=on  GotoTag=theta_b
  G1 : Subsystem  Commented=on
  G123 : Subsystem
  G123 {1..8} (8 alike) : Scope
  Gain : Gain  Gain=[1 1 1]
  Gain1 : Gain  Gain=-L
  Gain2 : Gain  Gain=L
  Gain3 : Gain
  Gain4 : Gain  Gain=[ 1 1 1]
  Ground : Ground
  IC : InitialCondition  Value=0
  M_12 : Subsystem  Commented=on
  M_123 : Subsystem
  Math Function : Math  Operator=square  SaturateOnIntegerOverflow=on
  Math Function1 : Math  Operator=transpose  SaturateOnIntegerOverflow=on
  Mux : Mux  Inputs=2
  Mux1 : Mux  Inputs=2
  Product1 : Product  Inputs=**  SaturateOnIntegerOverflow=on  InputSameDT=on  OutDataTypeStr=Inherit: Same as first input
  Product2 : Product  Inputs=**  SaturateOnIntegerOverflow=on  InputSameDT=on  OutDataTypeStr=Inherit: Same as first input
  Product3 : Product  Inputs=*/*  Multiplication=Matrix(*)  SaturateOnIntegerOverflow=on  InputSameDT=on  OutDataTypeStr=Inherit: Same as first input
  Product4 : Product  Inputs=**  Multiplication=Matrix(*)  SaturateOnIntegerOverflow=on  InputSameDT=on  OutDataTypeStr=Inherit: Same as first input
  Product5 : Product  Inputs=**  Multiplication=Matrix(*)  SaturateOnIntegerOverflow=on  InputSameDT=on  OutDataTypeStr=Inherit: Same as first input
  Product6 : Product  Multiplication=Matrix(*)
  Product8 : Product  Inputs=*/  SaturateOnIntegerOverflow=on  InputSameDT=on  OutDataTypeStr=Inherit: Same as first input
  Quadrotor Dynamics Outer-Loop : Subsystem
  Saturation : Saturate  UpperLimit=0.15  LowerLimit=-0.15
  Signal Specification1 : SignalSpecification  Dimensions=3
  Signal Specification2 : SignalSpecification  Dimensions=2
  Signal Specification3 : SignalSpecification  Dimensions=3
  Signal Specification5 : SignalSpecification  Dimensions=2
  Sum1 : Sum  Inputs=|+-
  Sum2 : Sum  Inputs=-+|  SaturateOnIntegerOverflow=on
  Sum3 : Sum  Inputs=|+-
  Sum4 : Sum  Inputs=-+|  SaturateOnIntegerOverflow=on
  Sum5 : Sum  Inputs=|-+  SaturateOnIntegerOverflow=on
  Sum6 : Sum  Inputs=-+|  SaturateOnIntegerOverflow=on
  "T, r,xu,xb" : Scope
  "Tension from Buoy, X direction" : Subsystem  Commented=on
  "Tension from UAV, X and r directions" : Subsystem
  Terminator : Terminator
  "V_im " : Scope
  V_im 1 : Scope
  V_im 3 : Scope
  Vector Concatenate{,1..2,4,6} (5 alike) : Concatenate
  Vector Concatenate10 : Concatenate  NumInputs=3
  Vector Concatenate5 : Concatenate  NumInputs=3
  "XZb ddot " : Scope
  "alpha  " : Scope
  azimuthal dynamics : Subsystem
  buoyancy : Subsystem
  ddotr_p1 : Selector  InputPortWidth=2  IndexOptions=Index vector (dialog)  Indices=1  OutputSizes=2
  dot(theta) : DiscreteIntegrator  gainval=1  InitialCondition=q_b_ini  SampleTime=-1  ICPrevOutput=DiscIntNeverNeededParam  ICPrevScaledInput=DiscIntNeverNeededParam
  dot(x,z,alpha) : DiscreteIntegrator  InitialCondition=[v_b_ini]  SampleTime=-1  ICPrevOutput=DiscIntNeverNeededParam  ICPrevScaledInput=DiscIntNeverNeededParam
  "is coupled " : Scope
  numerical error{,1..3} (4 alike) : Scope
  "rotation matrix R " : Subsystem
  theta : DiscreteIntegrator  InitialCondition=theta_q_ini  SampleTime=-1  StateName=theta  ICPrevOutput=DiscIntNeverNeededParam  ICPrevScaledInput=DiscIntNeverNeededParam
  theta u : Scope
  theta u1 : Scope
  u 1 : InportShadow
  "u1  " : InportShadow
  u123 : Subsystem
  x z ddot : Selector  InputPortWidth=3  IndexOptions=Index vector (dialog)  Indices=[1 2]  OutputSizes=1
  zeta1 : InportShadow  Port=3
  Xb : Outport  Unit=m  InitialOutput=0
  Xb_dot : Outport  Port=2  Unit=m  InitialOutput=0
  Xb_ddot : Outport  Port=3  Unit=m  InitialOutput=0
  Attitude_buoy : Outport  Port=4  Unit=rad/s^2  InitialOutput=0
  Xu : Outport  Port=5  Unit=m  InitialOutput=0
  Xu_dot : Outport  Port=6  Unit=m/s  InitialOutput=0
  Xu_ddot : Outport  Port=7  Unit=m/s  InitialOutput=0
  Attitude_quadrotor : Outport  Port=8  Unit=rad  InitialOutput=0
  q_quadrotor : Outport  Port=9  Unit=rad/s  InitialOutput=0
  alpha : Outport  Port=10  Unit=m  InitialOutput=0
  alpha_dot : Outport  Port=11  Unit=m  InitialOutput=0
  alpha_ddot : Outport  Port=12  Unit=m  InitialOutput=0
  "  r" : Outport  Port=13  Unit=m  InitialOutput=0
  "  rdot" : Outport  Port=14  Unit=m  InitialOutput=0
  "  rddot" : Outport  Port=15  Unit=m  InitialOutput=0
  Cable Tension : Outport  Port=16  Unit=rad/s^2  InitialOutput=0
  V_im : Outport  Port=17  Unit=m  InitialOutput=0
  "D_123 " : Outport  Port=18  Unit=m  InitialOutput=0
  coupled : Outport  Port=19  Unit=m  InitialOutput=0
  wires:
  u123/1(u123) -> G123 5/1, Add/1
  Product4/1 -> G123 7/1, Add/3
  [D_123] -> Product4/1
  Vector Concatenate1/1 -> [eta_dot_tilde_123], Product4/2  "tilde{dot(q)}_123"
  G123/1(G) -> G123 8/1, Add/4
  [alpha] -> Mux1/2, "alpha  "/1, alpha/1
  [theta_b] -> D_123/2(theta_b)
  D_123/1(D_123) -> [D_123]
  [theta_b] -> M_123/1(theta)
  [alpha] -> M_123/2(alpha)
  Demux1/2 -> [zb_dot], Vector Concatenate4/2  "zb dot"
  Demux1/1 -> [xb_dot], Vector Concatenate4/1  "xb dot"
  [xb_dot] -> Vector Concatenate2/1
  [zb_dot] -> Vector Concatenate2/2
  Vector Concatenate2/1 -> Sum2/2
  V_w/1 -> Sum2/1
  Sum2/1 -> Vector Concatenate1/1
  Sum4/1 -> Vector Concatenate1/2
  theta_w/1 -> Gain3/1
  dot(theta)/1 -> q_quadrotor/1, theta/1
  theta/1 -> [theta_u], theta u/1, Attitude_quadrotor/1
  Constant7/1 -> Product8/2
  u2/1 -> Product8/1
  [theta_u] -> u123/2(theta)
  [V_im] -> u123/3(V_im)
  [alpha] -> G123/1(alpha)
  Demux/1 -> [xb], Vector Concatenate/1
  Demux/2 -> [zb], Vector Concatenate/2
  M_123/1(M_123) -> G123 1/1, [M_123]
  Product8/1 -> dot(theta)/1  "ddot(theta)"
  [M_123] -> G123 3/1, Product3/2
  Constant/1 -> Product3/1  "ddot(x,z,alpha)"
  Product3/1 -> Gain/1  "ddot(xb,zb,alpha)"
  IC/1 -> Saturation/1
  [alpha] -> C_123/1("alpha ")
  [alpha_dot] -> C_123/2(alpha_dot)
  C_123/1(C_123) -> [C_123]
  Vector Concatenate5/1 -> Signal Specification1/1
  [xb_dot] -> Vector Concatenate5/1
  [zb_dot] -> Vector Concatenate5/2
  [alpha_dot] -> Vector Concatenate5/3
  [C_123] -> Product5/1
  Product5/1 -> [Coriolis], Gain4/1
  Gain/1 -> [X123_ddot], x z ddot/1
  [alpha] -> u123/4(alpha)
  [r_p_ddot] -> ddotr_p1/1
  [theta_u] -> "Tension from UAV, X and r directions"/3(theta_u)
  u 1/1 -> "Tension from UAV, X and r directions"/4(u1)
  [D_123] -> "D_123 "/1, "D_123   "/1, Display1/1
  [M_123] -> Display/1
  [C_123] -> Display2/1
  (x,z,alpha)/1 -> Signal Specification5/1
  [zb] -> buoyancy/1(z_b)
  zeta/1 -> buoyancy/2(zeta)
  From34/1 -> "Tension from Buoy, X direction"/1(alpha)
  D_12/1 -> "Tension from Buoy, X direction"/3(D12)
  buoyancy/1(V_im) -> "V_im "/1, V_im/1, [V_im]
  M_12/1(M_12) -> "Tension from Buoy, X direction"/2(M12)
  From37/1 -> D_12/1
  From44/1 -> "Tension from Buoy, X direction"/5(Xb_ddot)
  From32/1 -> "Tension from Buoy, X direction"/4(Vr,Wr)
  [XZb_ddot] -> "Tension from UAV, X and r directions"/5(Xb_ddot)
  G1/1(G) -> "Tension from Buoy, X direction"/6(G)
  From51/1 -> M_12/1(theta)
  x z ddot/1 -> Xb_ddot/1, "XZb ddot "/1, [XZb_ddot], dot(x,z,alpha)/1
  ddotr_p1/1 -> "Tension from UAV, X and r directions"/2(r_p_ddot)
  [XZu_ddot] -> "Tension from UAV, X and r directions"/6(Xu_ddot)
  FB/1(Out1) -> "Tension from Buoy, X direction"/7(FB)
  Vector Concatenate10/1 -> "T, r,xu,xb"/1
  "Tension from Buoy, X direction"/1(T x,z) -> Vector Concatenate10/3
  Gain2/1 -> Vector Concatenate6/2
  [R_W_to_Wp] -> Product6/1
  Vector Concatenate6/1 -> Sum3/2
  "rotation matrix R "/1(R) -> [R_Wp_to_W], Math Function1/1
  Product6/1 -> Sum3/1, numerical error1/1, [r_p_ddot]
  Gain1/1 -> Vector Concatenate6/1
  Math Function/1 -> Gain1/1
  Sum1/1 -> Signal Specification2/1
  [XZu_ddot] -> numerical error2/1, Sum1/1
  Math Function1/1 -> [R_W_to_Wp]
  Sum3/1 -> numerical error/1
  [XZb_ddot] -> numerical error3/1, Sum1/2
  [alpha] -> "rotation matrix R "/1(angle (rad))
  [alpha_dot] -> Math Function/1
  Saturation/1 -> G123 2/1, Attitude_buoy/1, [theta_b]
  Add/1 -> G123 4/1, Signal Specification3/1
  Gain3/1 -> IC/1
  Gain4/1 -> G123 6/1, Add/2
  Product2/1 -> Sum4/2
  Ground/1 -> Sum4/1
  [eta_dot_tilde_123] -> D_123/1(eta_dot_tilde)
  Sum5/1 -> D_123/3(dh)
  [zb] -> Sum5/1
  zeta1/1 -> Sum5/2
  [coupled] -> C_123/3(coupled)
  [coupled] -> M_123/3(coupled)
  [coupled] -> G123/2(coupled)
  u1/1 -> u123/1(u1)
  Signal Specification1/1 -> Product5/2
  Signal Specification2/1 -> Product6/2, [r_ddot]
  Signal Specification3/1 -> Product3/3
  Signal Specification5/1 -> [XZb], Mux1/1, Demux/1
  Quadrotor Dynamics Outer-Loop/1(Xu) -> Xu/1, [Xu]
  [coupled] -> Delay13/1
  "u1  "/1 -> Quadrotor Dynamics Outer-Loop/5(u1)
  [theta_u] -> Quadrotor Dynamics Outer-Loop/6(theta_u)
  Quadrotor Dynamics Outer-Loop/2(dot(Xu)) -> [XZu_dot], Xu_dot/1
  Product1/1 -> Delay2/1
  [coupled] -> u123/5(coupled)
  [alpha_dot] -> Product2/1
  [coupled] -> Product2/2
  [Xu] -> Delay/1
  azimuthal dynamics/1(re-couple) -> [re_couple]
  azimuthal dynamics/2(alpha) -> V_im 3/1, [alpha]
  azimuthal dynamics/3("alpha_dot ") -> [alpha_dot]
  azimuthal dynamics/4(alpha_ddot) -> alpha_ddot/1, [alpha_ddot]
  Delay/1 -> azimuthal dynamics/2(Xu)
  azimuthal dynamics/5("r ") -> "  r"/1, "  r   "/1, [r_uav_buoy]
  [X123] -> Delay11/1
  Delay3/1 -> azimuthal dynamics/3(Xb)
  [X123_ddot] -> Delay12/1
  [X123_dot] -> Delay7/1
  dot(x,z,alpha)/1 -> Mux/1, (x,z,alpha)/1, [XZb_dot], Demux1/1
  [alpha_dot] -> alpha_dot/1, Mux/2
  Mux/1 -> [X123_dot]
  Mux1/1 -> [X123]
  Vector Concatenate4/1 -> Xb_dot/1
  Vector Concatenate/1 -> Xb/1
  [alpha] -> "Tension from UAV, X and r directions"/1(alpha)
  [XZb] -> Delay3/1
  [XZu_dot] -> Delay4/1
  [XZb_dot] -> Delay5/1
  [XZu_ddot] -> Delay6/1
  [XZb_ddot] -> Delay8/1
  [alpha_ddot] -> Gain2/1
  Delay4/1 -> azimuthal dynamics/4("Xu_dot ")
  [X123_ddot] -> Delay9/1
  Delay5/1 -> azimuthal dynamics/5(Xb_dot)
  Delay6/1 -> azimuthal dynamics/6(Xu_ddot)
  Delay8/1 -> azimuthal dynamics/7("Xb_ddot   ")
  Delay9/1 -> azimuthal dynamics/8("X123_ddot  ")
  [coupled] -> Delay1/1
  Delay1/1 -> V_im 1/1, azimuthal dynamics/1(coupled)
  Delay11/1 -> Quadrotor Dynamics Outer-Loop/1(X123)
  Delay12/1 -> Quadrotor Dynamics Outer-Loop/3(Xddot123)
  Delay7/1 -> Quadrotor Dynamics Outer-Loop/2(Xdot123)
  Delay13/1 -> Quadrotor Dynamics Outer-Loop/4(coupled)
  azimuthal dynamics/6(r dot) -> "  rdot"/1, [rr_dot]
  azimuthal dynamics/7(r ddot) -> "  rddot"/1, [rr_ddot]
  "Tension from UAV, X and r directions"/2("T, from uav z") -> Coupling state/1(pos_T), Cable Tension/1, Vector Concatenate10/2
  [re_couple] -> Coupling state/2(re_couple)
  Coupling state/1(is coupled) -> "is coupled "/1, coupled/1, [coupled]
  Quadrotor Dynamics Outer-Loop/3(ddot(Xu)) -> Xu_ddot/1, theta u1/1, [XZu_ddot]
  Quadrotor Dynamics Outer-Loop/4(acc_b_u) -> Terminator/1
  "Tension from UAV, X and r directions"/1("T, from r") -> Vector Concatenate10/1
  D_u (vector for simplification)/1(Du) -> Product1/1
  [XZu_dot] -> Sum6/2
  Sum6/1 -> D_u (vector for simplification)/1(Vr), Product1/2
  Delay2/1 -> Quadrotor Dynamics Outer-Loop/7(Du)
  V_wind/1 -> Delay10/1
  Delay10/1 -> Sum6/1

== system Marine_LocoMotive_UAV/Save to file/mean absolute error ==
  In1 : Inport
  Abs : Abs
  Add : Sum
  Constant : Constant  Value=T
  Delay : Delay  DelayLength=1
  IC : InitialCondition
  Product1 : Product  Inputs=*/
  Product2 : Product  Inputs=*/
  Out1 : Outport
  wires:
  Product2/1 -> IC/1
  Add/1 -> Product1/1, Delay/1
  Delay/1 -> Add/1
  [time] -> Product2/1
  In1/1 -> Abs/1
  Product1/1 -> Out1/1
  Constant/1 -> Product2/2
  IC/1 -> Product1/2
  Abs/1 -> Add/2

== system Marine_LocoMotive_UAV/Scope/Subsystem ==
  In1 : Inport
  In2 : Inport  Port=2
  Product : Product
  Sqrt : Sqrt  SaturateOnIntegerOverflow=on
  Subtract : Sum  Inputs=+-
  Sum of Elements : Sum  Inputs=+
  Out1 : Outport
  wires:
  In1/1 -> Subtract/2
  Product/1 -> Sum of Elements/1
  Subtract/1 -> Product/2, Product/1
  In2/1 -> Subtract/1
  Sqrt/1 -> Out1/1, [r]
  Sum of Elements/1 -> Sqrt/1

== system Marine_LocoMotive_UAV/Scope/absolute mean ==
  u : Inport
  Abs : Abs
  Clock : Clock
  Current velocity : Scope
  Current velocity1 : Scope
  Current velocity2 : Scope
  Discrete-Time Integrator : DiscreteIntegrator  gainval=1  SampleTime=T  ICPrevOutput=DiscIntNeverNeededParam  ICPrevScaledInput=DiscIntNeverNeededParam
  Divide1 : Product  Inputs=*/
  mean : Outport
  wires:
  Discrete-Time Integrator/1 -> Current velocity1/1, Divide1/1
  Abs/1 -> Discrete-Time Integrator/1
  u/1 -> Current velocity/1, Abs/1
  Divide1/1 -> mean/1
  Clock/1 -> Current velocity2/1, Divide1/2

== system Marine_LocoMotive_UAV/Scope/absolute mean1 ==
  u : Inport
  Abs : Abs
  Clock : Clock
  Current velocity : Scope
  Current velocity1 : Scope
  Current velocity2 : Scope
  Discrete-Time Integrator : DiscreteIntegrator  gainval=1  SampleTime=T  ICPrevOutput=DiscIntNeverNeededParam  ICPrevScaledInput=DiscIntNeverNeededParam
  Divide1 : Product  Inputs=*/
  mean : Outport
  wires:
  Clock/1 -> Divide1/2, Current velocity2/1
  Divide1/1 -> mean/1
  u/1 -> Abs/1, Current velocity/1
  Abs/1 -> Discrete-Time Integrator/1
  Discrete-Time Integrator/1 -> Divide1/1, Current velocity1/1

== system Marine_LocoMotive_UAV/Sea/Single Wave ==
  note: Aw.Sin
  time : Inport
  x(t) : Inport  Port=2
  Constant : Constant  Value=epsilon
  Gain : Gain  Gain=omega
  Gain1 : Gain  Gain=k
  Gain2 : Gain  Gain=A
  Gain3 : Gain  Gain=omega*A
  Gain4 : Gain  Gain=omega*A
  Gain5 : Gain  Gain=A*k
  Sum : Sum  Inputs=++-
  Trigonometric Function : Trigonometry  Operator=sincos
  Trigonometric Function1 : Trigonometry  Operator=atan
  direction : Gain  Gain=w_dir
  direction1 : Gain  Gain=w_dir
  direction2 : Gain  Gain=w_dir
  zeta(x,t) : Outport
  theta_w(x,t) : Outport  Port=2
  u(z0,x,t) : Outport  Port=3
  w(z0,x,t) : Outport  Port=4
  wires:
  Gain/1 -> Sum/2
  Gain1/1 -> Sum/3
  x(t)/1 -> Gain1/1
  Trigonometric Function/1 -> Gain3/1, Gain2/1
  Constant/1 -> Sum/1
  time/1 -> direction/1
  direction/1 -> Gain/1
  Gain2/1 -> zeta(x,t)/1  "zeta(x,t)"
  Trigonometric Function/2 -> Gain5/1, Gain4/1
  Sum/1 -> Trigonometric Function/1
  Trigonometric Function1/1 -> theta_w(x,t)/1
  Gain5/1 -> Trigonometric Function1/1
  Gain3/1 -> direction1/1
  Gain4/1 -> direction2/1
  direction1/1 -> u(z0,x,t)/1
  direction2/1 -> w(z0,x,t)/1

== system Marine_LocoMotive_UAV/Sea/Single Wave1 ==
  note: Aw.Sin
  time : Inport
  x(t) : Inport  Port=2
  Constant : Constant  Value=epsilon
  Gain : Gain  Gain=omega
  Gain1 : Gain  Gain=k
  Gain2 : Gain  Gain=A
  Gain3 : Gain  Gain=omega*A
  Gain4 : Gain  Gain=omega*A
  Gain5 : Gain  Gain=A*k
  Sum : Sum  Inputs=++-
  Trigonometric Function : Trigonometry  Operator=sincos
  Trigonometric Function1 : Trigonometry  Operator=atan
  direction : Gain  Gain=w_dir
  direction1 : Gain  Gain=w_dir
  direction2 : Gain  Gain=w_dir
  zeta(x,t) : Outport
  theta_w(x,t) : Outport  Port=2
  u(z0,x,t) : Outport  Port=3
  w(z0,x,t) : Outport  Port=4
  wires:
  direction2/1 -> w(z0,x,t)/1
  direction1/1 -> u(z0,x,t)/1
  Gain4/1 -> direction2/1
  Gain3/1 -> direction1/1
  Gain5/1 -> Trigonometric Function1/1
  Trigonometric Function1/1 -> theta_w(x,t)/1
  Sum/1 -> Trigonometric Function/1
  Trigonometric Function/2 -> Gain4/1, Gain5/1
  Gain2/1 -> zeta(x,t)/1  "zeta(x,t)"
  direction/1 -> Gain/1
  time/1 -> direction/1
  Constant/1 -> Sum/1
  Trigonometric Function/1 -> Gain2/1, Gain3/1
  x(t)/1 -> Gain1/1
  Gain1/1 -> Sum/3
  Gain/1 -> Sum/2

== system Marine_LocoMotive_UAV/Sea/Theta_water surface (two waves) ==
  w1 : Inport
  w2 : Inport  Port=2
  Gain2 : Gain  Gain=1/(omega_w)
  Gain3 : Gain  Gain=k_w
  Gain4 : Gain  Gain=1/(omega_w2)
  Gain5 : Gain  Gain=k_w2
  Sum2 : Sum  Inputs=++|
  direction1 : Gain  Gain=1/w_dir
  direction2 : Gain  Gain=1/w_dir2
  Out1 : Outport
  wires:
  Gain4/1 -> direction2/1
  direction2/1 -> Gain5/1
  Sum2/1 -> Out1/1
  w1/1 -> Gain2/1
  Gain3/1 -> Sum2/1
  Gain5/1 -> Sum2/2
  w2/1 -> Gain4/1
  direction1/1 -> Gain3/1
  Gain2/1 -> direction1/1

== system Marine_LocoMotive_UAV/Sensors and Filters/Coupling detection by r ==
  In1 : Inport
  In2 : Inport  Port=2
  Constant1 : Constant  Value=0
  Coupling state : Subsystem
  Data Type Conversion : DataTypeConversion  OutDataTypeStr=double
  IC2 : InitialCondition  Value=0
  Switch14 : Switch  Criteria=u2 > Threshold  Threshold=0.5
  cable length with safety margine : simulink/Logic and Bit Operations/Compare To Constant  relop=>=  const=Lc_0+0.005  OutDataTypeStr=boolean
  is coupled {,2..4} (4 alike) : Scope
  is coupled : Outport
  wires:
  IC2/1 -> Switch14/3
  In1/1 -> is coupled 3/1, Coupling state/1(r_est), is coupled 2/1, cable length with safety margine/1
  Switch14/1 -> [re_couple]
  cable length with safety margine/1 -> is coupled 4/1, Data Type Conversion/1
  [re_couple] -> Coupling state/2(re_couple)
  Data Type Conversion/1 -> IC2/1
  Coupling state/1(is coupled) -> is coupled/1, "is coupled "/1
  Constant1/1 -> Switch14/1
  In2/1 -> Switch14/2

== system Marine_LocoMotive_UAV/Sensors and Filters/Data processing ==
  Acc : Inport
  "GPS " : Inport  Port=2
  p,q,r : Inport  Port=3
  Sonar : Inport  Port=4
  Estimate Attitude : Subsystem  TreatAsAtomicUnit=on  SystemSampleTime=Tc
  Estimate Position : Subsystem  TreatAsAtomicUnit=on  SystemSampleTime=Tc
  "Euler " : Selector  InputPortWidth=5  IndexOptions=Index vector (dialog)  Indices=[3]  OutputSizes=1
  GPS : InportShadow  Port=2
  Xe_est : Outport
  Ve_est : Outport  Port=2
  q_gyro : Outport  Port=3
  "q_est " : Outport  Port=4
  pitch_est : Outport  Port=5
  wires:
  GPS/1 -> "Euler "/1
  Acc/1 -> Estimate Attitude/1(Acc)
  p,q,r/1 -> Estimate Attitude/2(q)
  "Euler "/1 -> Estimate Attitude/3(Euler)
  Estimate Attitude/2(q_f) -> "q_est "/1
  "GPS "/1 -> Estimate Position/1(OptiTrack)
  Estimate Position/1(Xe) -> Xe_est/1
  Estimate Position/2(Ve) -> Ve_est/1
  Estimate Attitude/1(q_g) -> q_gyro/1
  Sonar/1 -> Estimate Position/3(Sonar)
  Estimate Attitude/3(" pitch") -> Estimate Position/2("pitch, Kalman"), pitch_est/1

== system Marine_LocoMotive_UAV/Sensors and Filters/GPS//INS ==
  X : Inport
  X_dot : Inport  Port=2
  X_ddot : Inport  Port=3
  q : Inport  Port=4
  theta : Inport  Port=5
  Discrete Derivative1 : simulink/Discrete/Discrete Derivative  gainval=1.0  ICPrevScaledInput=0.0  OutMin=[]  OutMax=[]  OutDataType=fixdt(1, 16)  OutScaling=2^-10  DoSatur=off
  Discrete Derivative2 : simulink/Discrete/Discrete Derivative  gainval=1.0  ICPrevScaledInput=0.0  OutMin=[]  OutMax=[]  OutDataType=fixdt(1, 16)  OutScaling=2^-10  DoSatur=off
  GPS noise : RandomNumber  Variance=5/10000  Seed=123  SampleTime=Tg
  Gain : Gain  Gain=0.25
  Gain1 : Gain  Gain=0.5
  Gain2 : Gain
  Gain3 : Gain
  Gain4 : Gain
  IMU noise : RandomNumber  Variance=1/10000  Seed=2235  SampleTime=Ts
  Low Pass Filter{1,3..5} (4 alike) : DiscreteTransferFcn  Numerator=Bm_LPF2  Denominator=Am_LPF2
  Low Pass Filter2 : DiscreteTransferFcn  Numerator=Bm_LPF  Denominator=Am_LPF
  Mux4 : Mux  Inputs=2
  Rate Transition : RateTransition
  Rate Transition1 : RateTransition
  Sum{1,3..6} (5 alike) : Sum  Inputs=++|
  q1 : Scope
  q2 : Scope
  q3 : Scope
  X_est : Outport
  X_dot_est : Outport  Port=2
  q_est : Outport  Port=3
  theta_est : Outport  Port=4
  X_ddot_est : Outport  Port=5
  wires:
  Sum4/1 -> X_dot_est/1
  Low Pass Filter1/1 -> Low Pass Filter3/1
  Gain3/1 -> Sum6/1
  q/1 -> Sum6/2
  theta/1 -> Sum5/2
  Gain2/1 -> Sum5/1
  Rate Transition1/1 -> Low Pass Filter2/1
  IMU noise/1 -> Rate Transition1/1
  Mux4/1 -> Gain1/1
  X/1 -> Sum3/2
  GPS noise/1 -> Rate Transition/1
  Rate Transition/1 -> Low Pass Filter1/1
  Sum5/1 -> theta_est/1
  X_dot/1 -> Sum4/2
  Sum3/1 -> X_est/1
  Sum6/1 -> q_est/1
  Low Pass Filter2/1 -> Gain3/1, Gain2/1, q2/1
  Low Pass Filter3/1 -> Mux4/2, Mux4/1
  Discrete Derivative1/1 -> Low Pass Filter4/1
  Gain1/1 -> Discrete Derivative1/1, Sum3/1, q1/1
  Gain/1 -> Discrete Derivative2/1, Sum4/1, q3/1
  Discrete Derivative2/1 -> Low Pass Filter5/1
  X_ddot/1 -> Sum1/2
  Gain4/1 -> Sum1/1
  Sum1/1 -> X_ddot_est/1
  Low Pass Filter4/1 -> Gain/1
  Low Pass Filter5/1 -> Gain4/1
